simulink model "AMCLIB_CurrentLoop_BAM_F32"  (Simulink 8.3)
settings: Solver=ode45  StartTime=0.0  StopTime=10.0  RelTol=1e-3
undefined symbols (not defined in the file): f32CC1scD, f32CC1scQ, f32CC2scD, f32CC2scQ, u16NShiftD, u16NShiftQ
settings Model: Creator=B37097  LastModifiedBy=B37097
settings DataIOCC: SignalLoggingSaveFormat=Dataset
settings DebuggingCC: UnderspecifiedInitializationDetection=Simplified  StateNameClashWarn=none
settings GRTTargetCC: CombineOutputUpdateFcns=on  GRTInterface=off

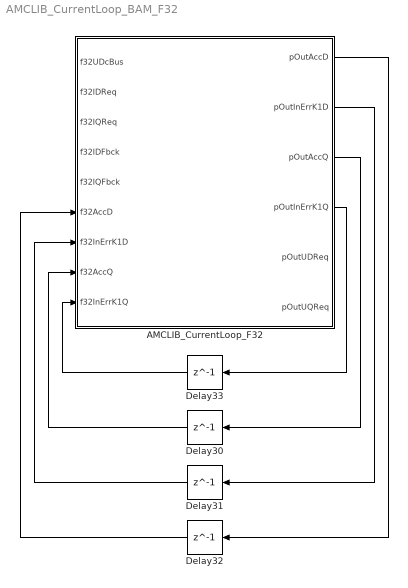
== system AMCLIB_CurrentLoop_BAM_F32 ==
  AMCLIB_CurrentLoop_F32 : Subsystem  mask(AMCLIB_CurrentLoop_F32){f32CC1scD=f32CC1scD, f32CC2scD=f32CC2scD, u16NShiftD=u16NShiftD, f32CC1scQ=f32CC1scQ, f32CC2scQ=f32CC2scQ, u16NShiftQ=u16NShiftQ}
      mask help: Bit accurate model of the current loop algorithm for a PMSM in 32-bit fixed-point implementation.
      mask init:
      | pos = get_param(gcb, 'Position');width = pos(3) - pos(1); height = pos(4) - pos(2);tX=width/2;tY=height*0.9;
      mask Display: color('black');port_label('input',1,'f32UDcBus');port_label('input',2,'f32IDReq');port_label('input',3,'f32IQReq');port_label('input',4,'f32IDFbck');port_label('input',5,'f32IQFbck');port_label('input',6,'f32AccD');port_label('input',7,'f32InErrK1D');port_label('input',8,'f32AccQ');port_label('input',9,'f32InErrK1Q');port_label('output',1,'pOutAccD');port_label('output',2,'pOutInErrK1D');port_label('output',3,'pOutAccQ');port_label('output',4,'pOutInErrK1Q');port_label('output',5,'pOutUDReq');port_label('output',6,'pOutUQReq');color('black');disp('AMCLIB_CurrentLoop_F32');color('blue');text(tX,tY, 'BAM', 'horizontalAlignment', 'center');
  Delay{30..33} (4 alike) : Delay  DelayLength=1  InitialCondition=0
  wires:
  AMCLIB_CurrentLoop_F32/4(pOutInErrK1Q) -> Delay33/1
  Delay33/1 -> AMCLIB_CurrentLoop_F32/9(f32InErrK1Q)
  AMCLIB_CurrentLoop_F32/3(pOutAccQ) -> Delay30/1
  Delay30/1 -> AMCLIB_CurrentLoop_F32/8(f32AccQ)
  AMCLIB_CurrentLoop_F32/2(pOutInErrK1D) -> Delay31/1
  Delay31/1 -> AMCLIB_CurrentLoop_F32/7(f32InErrK1D)
  AMCLIB_CurrentLoop_F32/1(pOutAccD) -> Delay32/1
  Delay32/1 -> AMCLIB_CurrentLoop_F32/6(f32AccD)

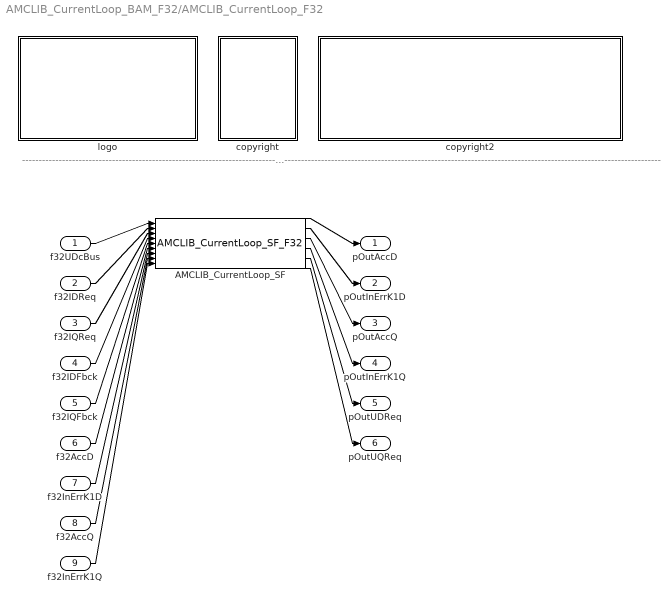
== system AMCLIB_CurrentLoop_BAM_F32/AMCLIB_CurrentLoop_F32 ==
  note: ---------------------------------------------------------------------------------------------------------------------------------------------------------------------------------------------------
  f32UDcBus : Inport
  f32IDReq : Inport  Port=2
  f32IQReq : Inport  Port=3
  f32IDFbck : Inport  Port=4
  f32IQFbck : Inport  Port=5
  f32AccD : Inport  Port=6
  f32InErrK1D : Inport  Port=7
  f32AccQ : Inport  Port=8
  f32InErrK1Q : Inport  Port=9
  AMCLIB_CurrentLoop_SF : S-Function  FunctionName=AMCLIB_CurrentLoop_SF_F32  Parameters=f32CC1scD,f32CC2scD,u16NShiftD,f32CC1scQ,f32CC2scQ,u16NShiftQ  EnableBusSupport=off
  copyright : Subsystem
      mask Display: text(10,90,'FILE:');text(10,75,'DESRIPTION:');text(10,60,'COPYRIGHT:');text(10,45,'VERSION:');text(10,30,'DATE:')
  copyright2 : Subsystem
      mask Display: text(10,90,'AMCLIB_CurrentLoop_BAM_F32.mdl');text(10,75,'PMSM Current Loop.');text(10,60,'NXP');text(10,45,'1.0');text(10,30,'25-Oct-2017');
  logo : Subsystem
      mask Display: image(imread('logo.jpg'))
  pOutAccD : Outport
  pOutInErrK1D : Outport  Port=2
  pOutAccQ : Outport  Port=3
  pOutInErrK1Q : Outport  Port=4
  pOutUDReq : Outport  Port=5
  pOutUQReq : Outport  Port=6
  wires:
  f32UDcBus/1 -> AMCLIB_CurrentLoop_SF/1
  f32IDReq/1 -> AMCLIB_CurrentLoop_SF/2
  f32IQReq/1 -> AMCLIB_CurrentLoop_SF/3
  f32IDFbck/1 -> AMCLIB_CurrentLoop_SF/4
  f32IQFbck/1 -> AMCLIB_CurrentLoop_SF/5
  f32AccD/1 -> AMCLIB_CurrentLoop_SF/6
  f32InErrK1D/1 -> AMCLIB_CurrentLoop_SF/7
  f32AccQ/1 -> AMCLIB_CurrentLoop_SF/8
  f32InErrK1Q/1 -> AMCLIB_CurrentLoop_SF/9
  AMCLIB_CurrentLoop_SF/1 -> pOutAccD/1
  AMCLIB_CurrentLoop_SF/2 -> pOutInErrK1D/1
  AMCLIB_CurrentLoop_SF/3 -> pOutAccQ/1
  AMCLIB_CurrentLoop_SF/4 -> pOutInErrK1Q/1
  AMCLIB_CurrentLoop_SF/5 -> pOutUDReq/1
  AMCLIB_CurrentLoop_SF/6 -> pOutUQReq/1

== system AMCLIB_CurrentLoop_BAM_F32/AMCLIB_CurrentLoop_F32/copyright ==

== system AMCLIB_CurrentLoop_BAM_F32/AMCLIB_CurrentLoop_F32/copyright2 ==

== system AMCLIB_CurrentLoop_BAM_F32/AMCLIB_CurrentLoop_F32/logo ==
